simulink model "BangBangABS"  (R2025b)
settings: configuration reference "VehicleFixed1ms" (kept outside this file)
libraries: simulink x4
settings Model: DataDictionary=VirtualMotoTemplate.sldd  ModifiedByFormat=The MathWorks, Inc.  Creator=The MathWorks, Inc.  LastModifiedBy=The MathWorks, Inc.
settings ConfigSetRef: SourceName=VehicleFixed1ms

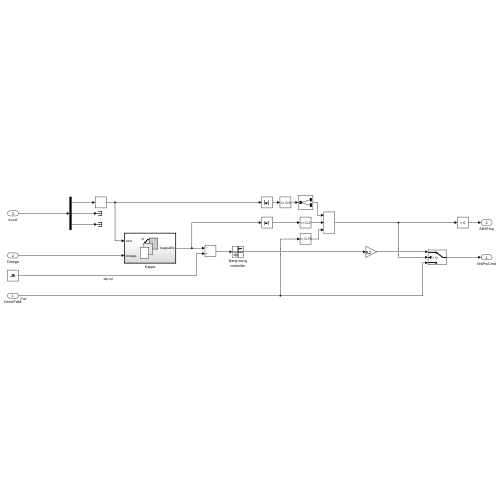
[thumbnail: Simulink's stored preview of the top-level diagram]
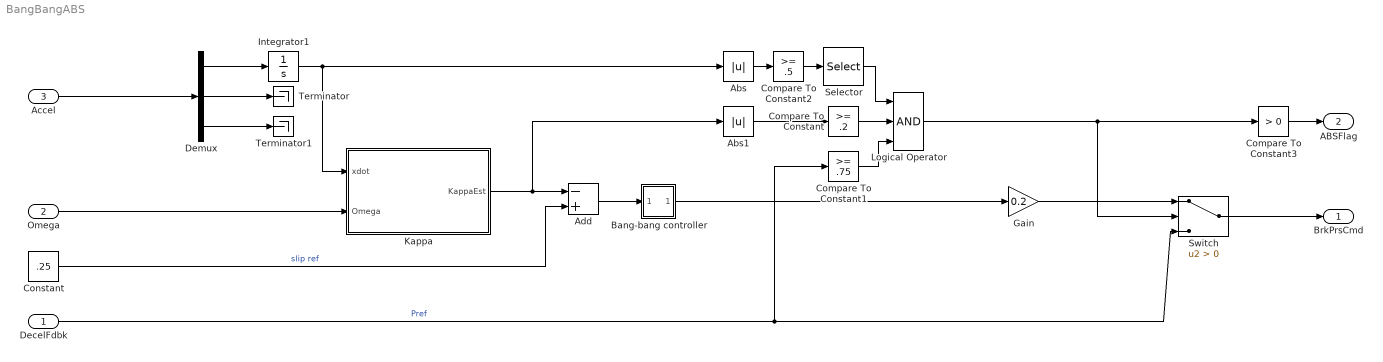
== system BangBangABS ==
  DecelFdbk : Inport  PortDimensions=2
  Omega : Inport  Port=2  PortDimensions=2
  Accel : Inport  Port=3
  Abs : Abs  SaturateOnIntegerOverflow=off
  Abs1 : Abs  SaturateOnIntegerOverflow=off
  Add : Sum  Inputs=-+
  Bang-bang controller : Subsystem  mask(Sign){}
      mask help: y = sign(x)
      mask Help: Sign Function:\n\t\t\ty = 1 if x > 0\n\t\t\ty = 0 if x = 0\n\t\t\ty = -1 if x < 0
      mask Display: plot(-50,-50,50,50,[-50,50],[0,0],[0,0],[-50,50],[-40,0],[-30,-30],[0,40],[30,30])
  Compare To Constant : simulink/Logic and Bit Operations/Compare To Constant  relop=>=  const=.2  OutDataTypeStr=boolean
  Compare To Constant1 : simulink/Logic and Bit Operations/Compare To Constant  relop=>=  const=.75  OutDataTypeStr=boolean
  Compare To Constant2 : simulink/Logic and Bit Operations/Compare To Constant  relop=>=  const=.5  OutDataTypeStr=boolean
  Compare To Constant3 : simulink/Logic and Bit Operations/Compare To Constant  relop=>  const=0  OutDataTypeStr=boolean  ZeroCross=off
  Constant : Constant  Value=.25
  Demux : Demux  Outputs=3
  Gain : Gain  Gain=0.2
  Integrator1 : Integrator
  Kappa : Subsystem  TreatAsAtomicUnit=on
  Logical Operator : Logic  Inputs=3  AllPortsSameDT=off  OutDataTypeStr=boolean
  Selector : Selector  InputPortWidth=1  IndexOptions=Index vector (dialog)  Indices=[1 1]  OutputSizes=1
  Switch : Switch  Criteria=u2 > Threshold  ZeroCross=off  SaturateOnIntegerOverflow=off  InputSameDT=off
  Terminator : Terminator
  Terminator1 : Terminator
  BrkPrsCmd : Outport  PortDimensions=2  VectorParamsAs1DForOutWhenUnconnected=off
  ABSFlag : Outport  Port=2  PortDimensions=2
  wires:
  Compare To Constant3/1 -> ABSFlag/1
  Abs1/1 -> Compare To Constant/1
  DecelFdbk/1 -> Compare To Constant1/1, Switch/3  "Pref"
  Omega/1 -> Kappa/2(Omega)
  Switch/1 -> BrkPrsCmd/1
  Demux/3 -> Terminator1/1
  Compare To Constant2/1 -> Selector/1
  Integrator1/1 -> Abs/1, Kappa/1(xdot)
  Demux/1 -> Integrator1/1
  Add/1 -> Bang-bang controller/1(in_1)
  Demux/2 -> Terminator/1
  Gain/1 -> Switch/1
  Kappa/1(KappaEst) -> Abs1/1, Add/1
  Accel/1 -> Demux/1
  Compare To Constant/1 -> Logical Operator/2
  Bang-bang controller/1(out_1) -> Gain/1
  Compare To Constant1/1 -> Logical Operator/3
  Constant/1 -> Add/2  "slip ref"
  Logical Operator/1 -> Switch/2, Compare To Constant3/1
  Abs/1 -> Compare To Constant2/1
  Selector/1 -> Logical Operator/1

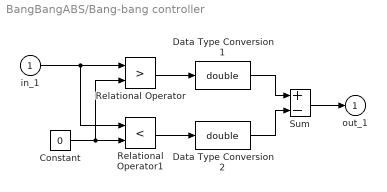
== system BangBangABS/Bang-bang controller ==
  in_1 : Inport
  Constant : Constant  Value=0
  Data Type Conversion1 : DataTypeConversion  OutDataTypeStr=double
  Data Type Conversion2 : DataTypeConversion  OutDataTypeStr=double
  Relational Operator : RelationalOperator  Operator=>  OutDataTypeStr=boolean
  Relational Operator1 : RelationalOperator  Operator=<  OutDataTypeStr=boolean
  Sum : Sum  Inputs=+-  InputSameDT=on  SaturateOnIntegerOverflow=on  OutDataTypeStr=Inherit: Same as first input
  out_1 : Outport  InitialOutput=0  VectorParamsAs1DForOutWhenUnconnected=off
  wires:
  in_1/1 -> Relational Operator/1, Relational Operator1/1
  Constant/1 -> Relational Operator1/2, Relational Operator/2
  Relational Operator1/1 -> Data Type Conversion2/1
  Relational Operator/1 -> Data Type Conversion1/1
  Sum/1 -> out_1/1
  Data Type Conversion1/1 -> Sum/1
  Data Type Conversion2/1 -> Sum/2

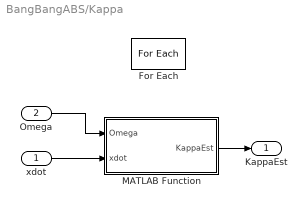
== system BangBangABS/Kappa ==
  xdot : Inport
  Omega : Inport  Port=2  Partition=on  PartitionDimension=1  PartitionWidth=1  PartitionOffset=0
  For Each : ForEach  DisableCoverage=on
  MATLAB Function : MATLAB Function  TreatAsAtomicUnit=on
  KappaEst : Outport  ConcatenationDimension=1
  wires:
  Omega/1 -> MATLAB Function/1(Omega)
  xdot/1 -> MATLAB Function/2(xdot)
  MATLAB Function/1(KappaEst) -> KappaEst/1

== matlab function BangBangABS/Kappa/MATLAB Function ==
  data: Omega input; xdot input; KappaEst output
function KappaEst = fcn(Omega, xdot)

Re = 0.29;
KappaEst = 0;
WhlSpd = Omega * Re;

if xdot*WhlSpd ~= 0
    KappaEst = (WhlSpd - xdot)/max([abs(xdot) abs(WhlSpd)]);
end
